simulink model "Smart_braking_logic"  (R2023b)
settings: Solver=ode3  StartTime=0.0  StopTime=180  FixedStep=0.1  RelTol=1e-3  EnableMultiTasking=on
model workspace (MAT data in the model file):
  A = Simulink.Parameter
  A.Value = 2.4
  A.DataType = 'auto'
  A.Complexity = 'real'
  A.Dimensions = [1 1]
  Cd = Simulink.Parameter
  Cd.Value = 0.32
  Cd.DataType = 'auto'
  Cd.Complexity = 'real'
  Cd.Dimensions = [1 1]
  Cr = Simulink.Parameter
  Cr.Value = 0.01
  Cr.DataType = 'auto'
  Cr.Complexity = 'real'
  Cr.Dimensions = [1 1]
  Tm = Simulink.Parameter
  Tm.Value = 190
  Tm.DataType = 'auto'
  Tm.Complexity = 'real'
  Tm.Dimensions = [1 1]
  betac = Simulink.Parameter
  betac.Value = 0.4
  betac.DataType = 'auto'
  betac.Complexity = 'real'
  betac.Dimensions = [1 1]
  g = Simulink.Parameter
  g.Value = 9.8
  g.DataType = 'auto'
  g.Complexity = 'real'
  g.Dimensions = [1 1]
  m = Simulink.Parameter
  m.Value = 1000
  m.DataType = 'auto'
  m.Complexity = 'real'
  m.Dimensions = [1 1]
  omegam = Simulink.Parameter
  omegam.Value = 420
  omegam.DataType = 'auto'
  omegam.Complexity = 'real'
  omegam.Dimensions = [1 1]
  rho = Simulink.Parameter
  rho.Value = 1.2
  rho.DataType = 'auto'
  rho.Complexity = 'real'
  rho.Dimensions = [1 1]
values from neighbouring files (symbols this model uses):
  g = gpuDevice    [Data_2.m]
libraries: simulink_extras x1, simulink x1
settings Model: Creator=root  LastModifiedBy=adity
settings SolverCC: ShapePreserveControl=EnableAll  AlgebraicLoopSolver=TrustRegion
settings OptimizationCC: DefaultUnderspecifiedDataType=single  EfficientFloat2IntCast=on  LifeSpan=inf
settings DebuggingCC: UnconnectedInputMsg=warning  UnconnectedOutputMsg=warning  UnconnectedLineMsg=warning  SFUnexpectedBacktrackingDiag=warning  SFNoUnconditionalDefaultTransitionDiag=warning  SFExecutionAtInitializationDiag=none  ArithmeticOperatorsInVariantConditions=warning
settings HardwareCC: ProdBitPerSizeT=32  ProdBitPerPtrDiffT=32  ProdWordSize=32  ProdHWDeviceType=Specified
settings ModelReferenceCC: EnableRefExpFcnMdlSchedulingChecks=on  PropagateSignalLabelsOutOfModel=off
settings SFSimCC: SimUseLocalCustomCode=off  CustomCodeUndefinedFunction=UseInterfaceOnly
settings RTWCC: RTWUseLocalCustomCode=off
settings CodeAppCC: StateflowObjectComments=on
settings GRTTargetCC: TargetLangStandard=C89/C90 (ANSI)
settings ConfigComp: CovMetricSettings=dw  CovSaveCumulativeToWorkspaceVar=on  CovSaveSingleToWorkspaceVar=on  CovExternalEMLEnable=off
settings SimscapeCC: SimscapeNormalizeSystem=off
settings ConfigurationSet: Description=SimMechanics 2G

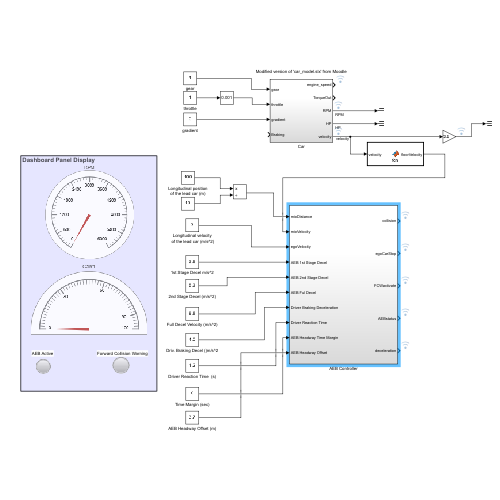
[thumbnail: Simulink's stored preview of the top-level diagram]
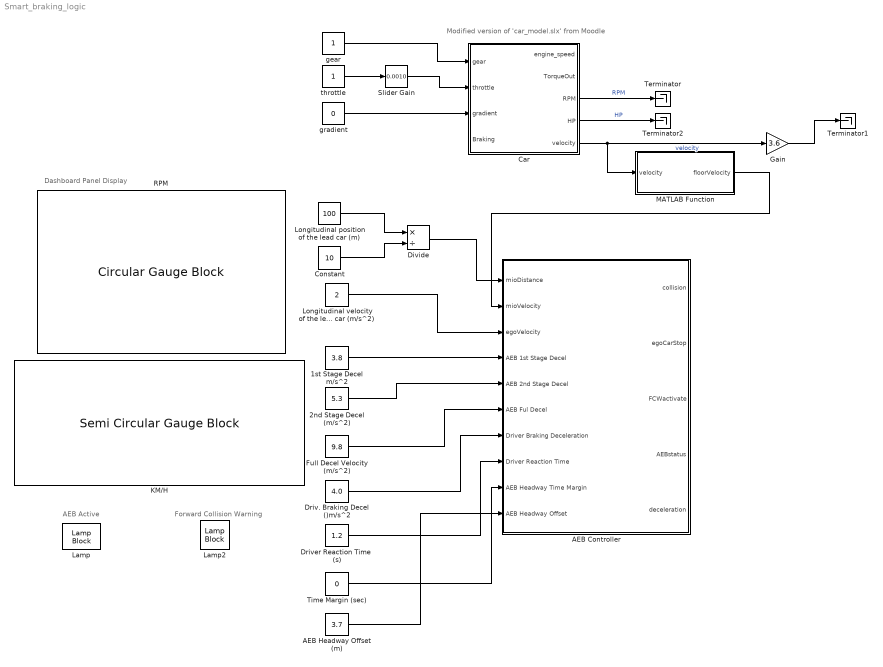
== system Smart_braking_logic ==
  note: Forward Collision Warning
  note: AEB Active
  note: Modified version of 'car_model.slx' from Moodle
  note: Dashboard Panel Display
  1st Stage Decel m/s^2 : Constant  Value=3.8
  2nd Stage Decel (m/s^2) : Constant  Value=5.3
  AEB Controller : Subsystem
  AEB Headway Offset (m) : Constant  Value=3.7
  Car : Subsystem
  Constant : Constant  Value=10
  Divide : Product  Inputs=*/
  Driv. Braking Decel ()m/s^2 : Constant  Value=4.0
  Driver Reaction Time  (s) : Constant  Value=1.2
  Full Decel Velocity (m/s^2) : Constant  Value=9.8
  Gain : Gain  Gain=3.6  OutMin=0
  KM/H : SemiCircularGaugeBlock  TickInterval=30
  Lamp : LampBlock  LabelPosition=Hide
  Lamp2 : LampBlock  LabelPosition=Hide
  Longitudinal position of the lead car (m) : Constant  Value=100
  Longitudinal velocity of the lead car (m/s^2) : Constant  Value=2
  MATLAB Function : MATLAB Function  TreatAsAtomicUnit=on
  RPM : CircularGaugeBlock  ScaleMax=6000
  Slider Gain : simulink/Math Operations/Slider Gain  gain=0.0010  low=0.001  high=1.1
  Terminator : Terminator
  Terminator1 : Terminator
  Terminator2 : Terminator
  Time Margin (sec) : Constant  Value=0
  gear : Constant
  gradient : Constant  Value=0
  throttle : Constant
  wires:
  Car/5(velocity) -> Gain/1, MATLAB Function/1(velocity)  "velocity"
  Car/3(RPM) -> Terminator/1  "RPM"
  Gain/1 -> Terminator1/1
  Car/4(HP) -> Terminator2/1  "HP"
  gear/1 -> Car/1(gear)
  gradient/1 -> Car/3(gradient)
  throttle/1 -> Slider Gain/1
  Slider Gain/1 -> Car/2(throttle)
  Time Margin (sec)/1 -> AEB Controller/9(AEB Headway Time Margin)
  Driver Reaction Time  (s)/1 -> AEB Controller/8(Driver Reaction Time)
  Driv. Braking Decel ()m/s^2/1 -> AEB Controller/7(Driver Braking Deceleration)
  Full Decel Velocity (m/s^2)/1 -> AEB Controller/6(AEB Ful Decel)
  2nd Stage Decel (m/s^2)/1 -> AEB Controller/5("AEB 2nd Stage Decel ")
  1st Stage Decel m/s^2/1 -> AEB Controller/4(AEB 1st Stage Decel)
  AEB Headway Offset (m)/1 -> AEB Controller/10(AEB Headway Offset)
  Longitudinal velocity of the lead car (m/s^2)/1 -> AEB Controller/3(egoVelocity)
  Divide/1 -> AEB Controller/1(mioDistance)
  Longitudinal position of the lead car (m)/1 -> Divide/1
  Constant/1 -> Divide/2
  MATLAB Function/1(floorVelocity) -> AEB Controller/2(mioVelocity)

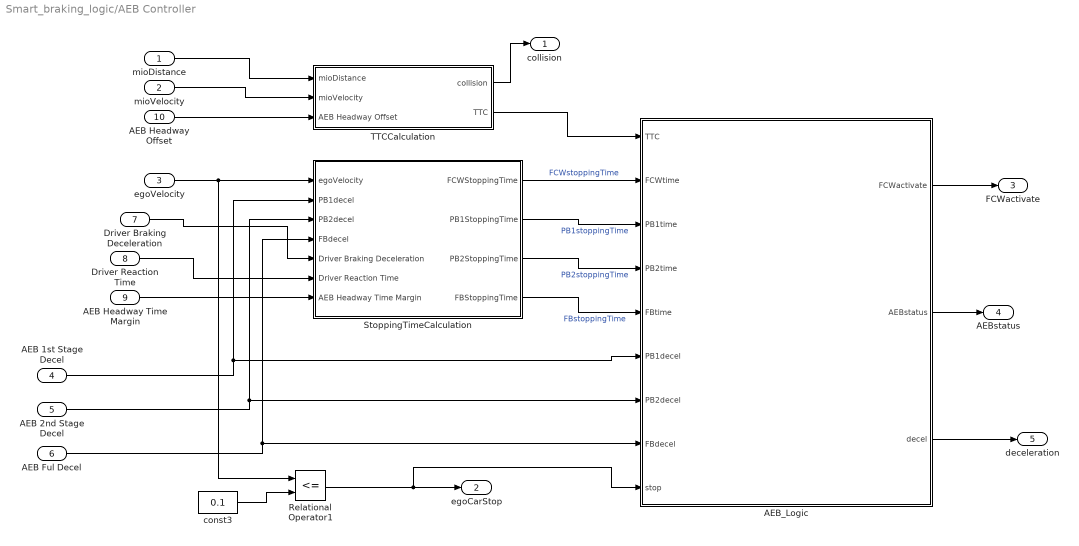
== system Smart_braking_logic/AEB Controller ==
  mioDistance : Inport
  mioVelocity : Inport  Port=2
  egoVelocity : Inport  Port=3
  AEB 1st Stage Decel : Inport  Port=4
  "AEB 2nd Stage Decel " : Inport  Port=5
  AEB Ful Decel : Inport  Port=6
  Driver Braking Deceleration : Inport  Port=7
  Driver Reaction Time : Inport  Port=8
  AEB Headway Time Margin : Inport  Port=9
  AEB Headway Offset : Inport  Port=10
  AEB_Logic : Stateflow chart  TreatAsAtomicUnit=on
  Relational Operator1 : RelationalOperator  Operator=<=  OutDataTypeStr=boolean  RndMeth=Simplest  InputSameDT=off
  StoppingTimeCalculation : Subsystem
  TTCCalculation : Subsystem
  const3 : Constant  Value=0.1  SampleTime=-1
  collision : Outport  VectorParamsAs1DForOutWhenUnconnected=off
  egoCarStop : Outport  Port=2  VectorParamsAs1DForOutWhenUnconnected=off
  FCWactivate : Outport  Port=3  VectorParamsAs1DForOutWhenUnconnected=off
  AEBstatus : Outport  Port=4  VectorParamsAs1DForOutWhenUnconnected=off
  deceleration : Outport  Port=5  VectorParamsAs1DForOutWhenUnconnected=off
  wires:
  AEB_Logic/3(decel) -> deceleration/1
  egoVelocity/1 -> Relational Operator1/1, StoppingTimeCalculation/1(egoVelocity)
  "AEB 2nd Stage Decel "/1 -> StoppingTimeCalculation/3(PB2decel), AEB_Logic/7(PB2decel)
  AEB Ful Decel/1 -> StoppingTimeCalculation/4(FBdecel), AEB_Logic/8(FBdecel)
  AEB_Logic/2(AEBstatus) -> AEBstatus/1
  const3/1 -> Relational Operator1/2
  Relational Operator1/1 -> AEB_Logic/9(stop), egoCarStop/1
  AEB 1st Stage Decel/1 -> StoppingTimeCalculation/2(PB1decel), AEB_Logic/6(PB1decel)
  StoppingTimeCalculation/3(PB2StoppingTime) -> AEB_Logic/4(PB2time)  "PB2stoppingTime"
  StoppingTimeCalculation/2(PB1StoppingTime) -> AEB_Logic/3(PB1time)  "PB1stoppingTime"
  StoppingTimeCalculation/4(FBStoppingTime) -> AEB_Logic/5(FBtime)  "FBstoppingTime"
  StoppingTimeCalculation/1(FCWStoppingTime) -> AEB_Logic/2(FCWtime)  "FCWstoppingTime"
  AEB_Logic/1(FCWactivate) -> FCWactivate/1
  mioDistance/1 -> TTCCalculation/1(mioDistance)
  mioVelocity/1 -> TTCCalculation/2(mioVelocity)
  TTCCalculation/1(collision) -> collision/1
  TTCCalculation/2(TTC) -> AEB_Logic/1(TTC)
  Driver Braking Deceleration/1 -> StoppingTimeCalculation/5(Driver Braking Deceleration)
  Driver Reaction Time/1 -> StoppingTimeCalculation/6(Driver Reaction Time)
  AEB Headway Time Margin/1 -> StoppingTimeCalculation/7(AEB Headway Time Margin)
  AEB Headway Offset/1 -> TTCCalculation/3(AEB Headway Offset)

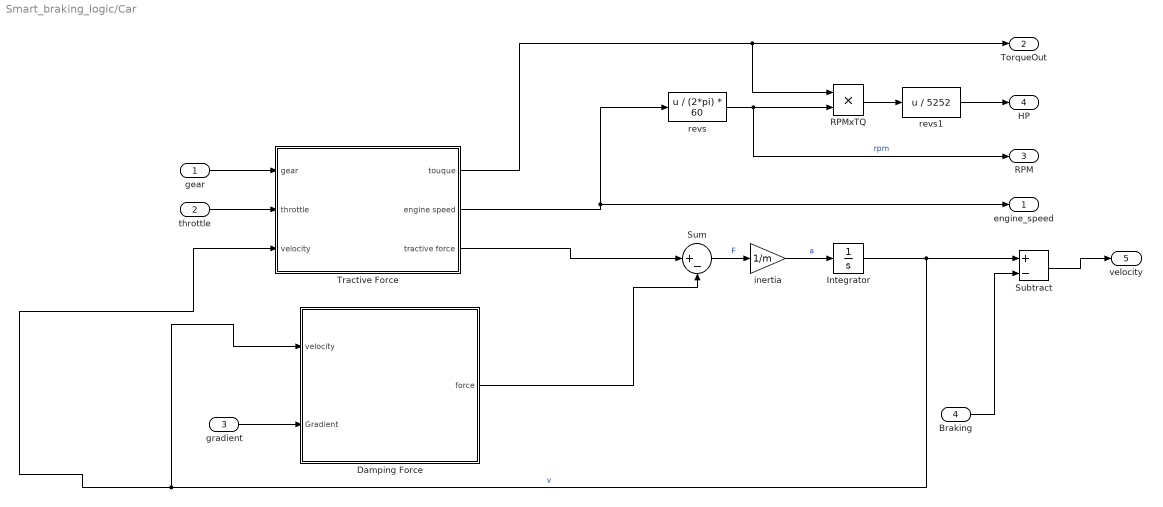
== system Smart_braking_logic/Car ==
  gear : Inport
  throttle : Inport  Port=2  OutMin=0  OutMax=1
  gradient : Inport  Port=3
  Braking : Inport  Port=4
  Damping Force : Subsystem
  Integrator : Integrator
  RPMxTQ : Product
  Subtract : Sum  Inputs=+-  OutMin=0  RndMeth=Round  SaturateOnIntegerOverflow=on
  Sum : Sum  Inputs=|+-
  Tractive Force : Subsystem
  inertia : Gain  Gain=1/m
  revs : Fcn  Expr=u / (2*pi) * 60
  revs1 : Fcn  Expr=u / 5252
  engine_speed : Outport  VectorParamsAs1DForOutWhenUnconnected=off
  TorqueOut : Outport  Port=2  VectorParamsAs1DForOutWhenUnconnected=off
  RPM : Outport  Port=3  VectorParamsAs1DForOutWhenUnconnected=off
  HP : Outport  Port=4  VectorParamsAs1DForOutWhenUnconnected=off
  velocity : Outport  Port=5  VectorParamsAs1DForOutWhenUnconnected=off
  wires:
  inertia/1 -> Integrator/1  "a"
  Sum/1 -> inertia/1  "F"
  Integrator/1 -> Subtract/1, Tractive Force/3(velocity), Damping Force/1(velocity)  "v"
  revs/1 -> RPM/1, RPMxTQ/2  "rpm"
  RPMxTQ/1 -> revs1/1
  revs1/1 -> HP/1
  Tractive Force/2(engine speed) -> revs/1, engine_speed/1
  Tractive Force/1(touque) -> TorqueOut/1, RPMxTQ/1
  gear/1 -> Tractive Force/1(gear)
  throttle/1 -> Tractive Force/2(throttle)
  Tractive Force/3(tractive force) -> Sum/1
  gradient/1 -> Damping Force/2(Gradient)
  Damping Force/1(force) -> Sum/2
  Subtract/1 -> velocity/1
  Braking/1 -> Subtract/2

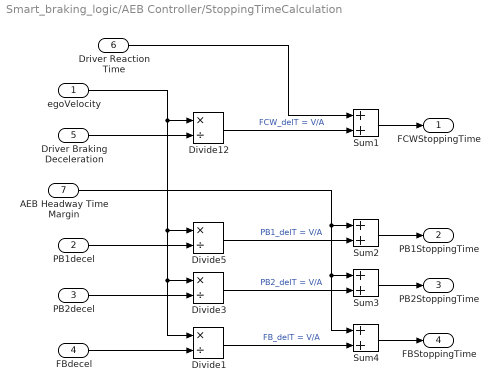
== system Smart_braking_logic/AEB Controller/StoppingTimeCalculation ==
  egoVelocity : Inport
  PB1decel : Inport  Port=2
  PB2decel : Inport  Port=3
  FBdecel : Inport  Port=4
  Driver Braking Deceleration : Inport  Port=5
  Driver Reaction Time : Inport  Port=6
  AEB Headway Time Margin : Inport  Port=7
  Divide{1,3,5,12} (4 alike) : Product  Inputs=*/
  Sum{1..4} (4 alike) : Sum
  FCWStoppingTime : Outport  VectorParamsAs1DForOutWhenUnconnected=off
  PB1StoppingTime : Outport  Port=2  VectorParamsAs1DForOutWhenUnconnected=off
  PB2StoppingTime : Outport  Port=3  VectorParamsAs1DForOutWhenUnconnected=off
  FBStoppingTime : Outport  Port=4  VectorParamsAs1DForOutWhenUnconnected=off
  wires:
  Sum1/1 -> FCWStoppingTime/1
  Sum2/1 -> PB1StoppingTime/1
  Sum3/1 -> PB2StoppingTime/1
  AEB Headway Time Margin/1 -> Sum2/1, Sum4/1, Sum3/1
  egoVelocity/1 -> Divide1/1, Divide3/1, Divide5/1, Divide12/1
  Divide5/1 -> Sum2/2  "PB1_delT = V/A"
  Divide3/1 -> Sum3/2  "PB2_delT = V/A"
  Divide1/1 -> Sum4/2  "FB_delT = V/A"
  Driver Braking Deceleration/1 -> Divide12/2
  PB1decel/1 -> Divide5/2
  PB2decel/1 -> Divide3/2
  FBdecel/1 -> Divide1/2
  Divide12/1 -> Sum1/2  "FCW_delT = V/A"
  Driver Reaction Time/1 -> Sum1/1
  Sum4/1 -> FBStoppingTime/1

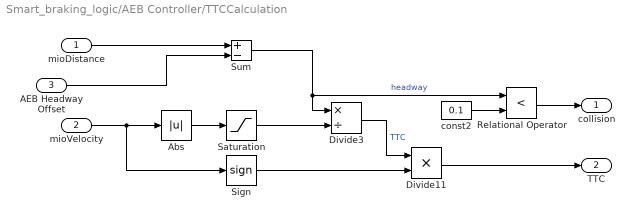
== system Smart_braking_logic/AEB Controller/TTCCalculation ==
  mioDistance : Inport
  mioVelocity : Inport  Port=2
  AEB Headway Offset : Inport  Port=3
  Abs : Abs  SaturateOnIntegerOverflow=off
  Divide11 : Product  Inputs=**
  Divide3 : Product  Inputs=*/
  Relational Operator : RelationalOperator  Operator=<  OutDataTypeStr=boolean  RndMeth=Simplest  InputSameDT=off
  Saturation : Saturate  UpperLimit=100  LowerLimit=0.01
  Sign : Signum
  Sum : Sum  Inputs=+-
  const2 : Constant  Value=0.1  SampleTime=-1
  collision : Outport  VectorParamsAs1DForOutWhenUnconnected=off
  TTC : Outport  Port=2  VectorParamsAs1DForOutWhenUnconnected=off
  wires:
  mioVelocity/1 -> Sign/1, Abs/1
  mioDistance/1 -> Sum/1
  Divide3/1 -> Divide11/1  "TTC"
  Sum/1 -> Relational Operator/1, Divide3/1  "headway"
  const2/1 -> Relational Operator/2
  Abs/1 -> Saturation/1
  Relational Operator/1 -> collision/1
  Saturation/1 -> Divide3/2
  Sign/1 -> Divide11/2
  Divide11/1 -> TTC/1
  AEB Headway Offset/1 -> Sum/2

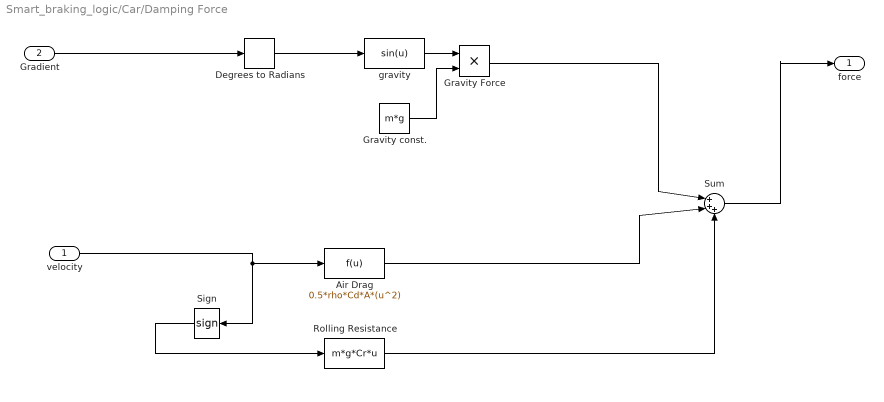
== system Smart_braking_logic/Car/Damping Force ==
  velocity : Inport
  Gradient : Inport  Port=2
  Air Drag : Fcn  Expr=0.5*rho*Cd*A*(u^2)
  Degrees to Radians : simulink_extras/Transformations/Degrees to Radians
  Gravity Force : Product
  Gravity const. : Constant  Value=m*g
  Rolling Resistance : Fcn  Expr=m*g*Cr*u
  Sign : Signum
  Sum : Sum  Inputs=|+++
  gravity : Fcn  Expr=sin(u)
  force : Outport  VectorParamsAs1DForOutWhenUnconnected=off
  wires:
  Sign/1 -> Rolling Resistance/1
  Rolling Resistance/1 -> Sum/3
  Gravity const./1 -> Gravity Force/2
  Gradient/1 -> Degrees to Radians/1
  Degrees to Radians/1 -> gravity/1
  gravity/1 -> Gravity Force/1
  Air Drag/1 -> Sum/2
  Gravity Force/1 -> Sum/1
  velocity/1 -> Air Drag/1, Sign/1
  Sum/1 -> force/1

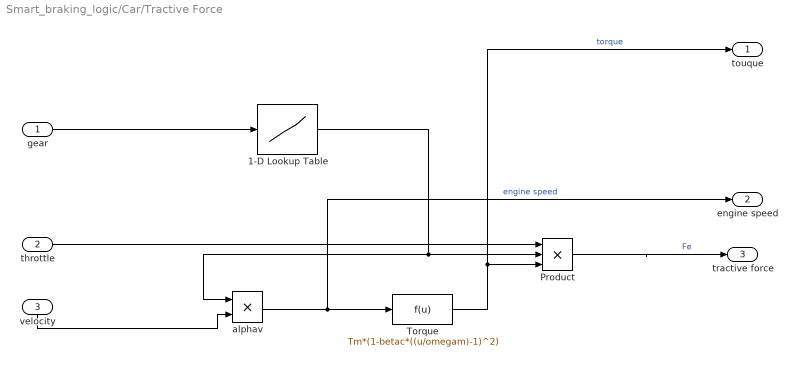
== system Smart_braking_logic/Car/Tractive Force ==
  gear : Inport
  throttle : Inport  Port=2
  velocity : Inport  Port=3
  1-D Lookup Table : Lookup_n-D  NumberOfTableDimensions=1  BreakpointsForDimension1=int16([1,2,3,4,5]);  Table=int16([40,25,16,12,10]);  InternalRulePriority=Speed  RndMeth=Simplest
  Product : Product  Inputs=3
  Torque : Fcn  Expr=Tm*(1-betac*((u/omegam)-1)^2)
  alphav : Product
  touque : Outport  VectorParamsAs1DForOutWhenUnconnected=off
  engine speed : Outport  Port=2  VectorParamsAs1DForOutWhenUnconnected=off
  tractive force : Outport  Port=3  VectorParamsAs1DForOutWhenUnconnected=off
  wires:
  gear/1 -> 1-D Lookup Table/1
  Torque/1 -> touque/1, Product/3  "torque"
  throttle/1 -> Product/1
  1-D Lookup Table/1 -> Product/2, alphav/1
  alphav/1 -> engine speed/1, Torque/1  "engine speed"
  Product/1 -> tractive force/1  "Fe"
  velocity/1 -> alphav/2

== matlab function Smart_braking_logic/MATLAB Function ==
  data: velocity input; floorVelocity output
function floorVelocity = fcn(velocity)
if velocity<0
    floorVelocity = 0;
else
    floorVelocity = velocity;
end

== stateflow chart Smart_braking_logic/AEB Controller/AEB_Logic ==
  note: FCW/AEB Logic
  state Default
    entry: AEBstatus = 0;
    FCWactivate = 0;
    decel = 0;
  state FCW
    entry: AEBstatus = 0;
    FCWactivate = 1;
    decel = 0;
  state Partial_Braking1
    entry: AEBstatus = 1;
    FCWactivate = 1;
    decel = PB1decel;
  state Full_Braking
    entry: AEBstatus = 3;
    FCWactivate = 1;
    decel = FBdecel;
  state Partial_Braking2
    entry: AEBstatus = 2;
    FCWactivate = 1;
    decel = PB2decel;
  (default) -> Default
  Full_Braking -> Default : [stop==1]
  Partial_Braking2 -> Default [order 2] : [stop==1]
  Partial_Braking1 -> Default [order 2] : [stop==1]
  Default -> FCW : [(abs(TTC)<FCWtime) && TTC<0]
  FCW -> Default [order 2] : [abs(TTC)>=1.2*FCWtime]
  FCW -> Partial_Braking1 [order 1] : [(abs(TTC) < PB1time) && TTC<0]
  Partial_Braking1 -> Partial_Braking2 [order 1] : [(abs(TTC) < PB2time) && TTC<0]
  Partial_Braking2 -> Full_Braking [order 1] : [(abs(TTC) < FBtime) && TTC<0]
  data: FCWactivate output; TTC input; FCWtime input; PB1time input; PB2time input; FBtime input; PB1decel input; PB2decel input; FBdecel input; AEBstatus output; decel output; stop input
